simulink model "control_system"  (R2019b)
settings: Solver=FixedStepAuto  StartTime=0.0  StopTime=10.0  RelTol=1e-3
undefined symbols (not defined in the file): thrust_lower_limit, thrust_upper_limit
settings Model: Creator=logan  LastModifiedBy=loganfillo
settings OptimizationCC: DefaultParameterBehavior=Inlined  UseDivisionForNetSlopeComputation=on  GainParamInheritBuiltInType=on  UseFloatMulNetSlope=on  InlineInvariantSignals=on  PassReuseOutputArgsAs=Individual arguments  ZeroExternalMemoryAtStartup=off  ZeroInternalMemoryAtStartup=off  NoFixptDivByZeroProtection=on  EfficientFloat2IntCast=on  LifeSpan=1  OptimizeBlockOrder=speed  DifferentSizesBufferReuse=on  EfficientTunableParamExpr=on
settings DebuggingCC: ParameterTunabilityLossMsg=error
settings HardwareCC: ProdLongLongMode=on
settings SFSimCC: MATLABDynamicMemAlloc=off
settings RTWCC: SystemTargetFile=ert.tlc  PackageGeneratedCodeAndArtifacts=on  TemplateMakefile=ert_default_tmf  GenerateReport=on  IncludeHyperlinkInReport=on  LaunchReport=on  TargetLang=C++  GenerateTraceInfo=on  GenerateTraceReport=on  GenerateTraceReportSl=on  GenerateTraceReportSf=on  GenerateTraceReportEml=on
settings CodeAppCC: ForceParamTrailComments=on  IgnoreCustomStorageClasses=off  OperatorAnnotations=on  SimulinkDataObjDesc=on  SFDataObjDesc=on  InsertBlockDesc=on
settings ERTTargetCC: TargetLangStandard=C++03 (ISO)  GenerateSampleERTMain=on  IncludeMdlTerminateFcn=off  CombineSignalStateStructs=on  MultiInstanceERTCode=on  CodeInterfacePackaging=C++ class  SupportComplex=off  SupportContinuousTime=on  InlinedParameterPlacement=NonHierarchical  RootIOFormat=Structure reference  ERTCustomFileTemplate=example_file_process.tlc  ERTFilePackagingFormat=CompactWithDataFile

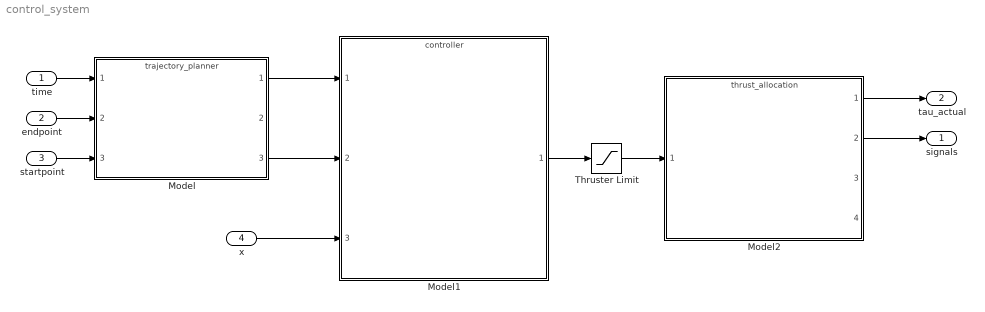
== system control_system ==
  "time " : Inport
  "endpoint " : Inport  Port=2  PortDimensions=6
  startpoint : Inport  Port=3  PortDimensions=6
  x : Inport  Port=4
  Model : ModelReference  ModelNameDialog=trajectory_planner.slx  SimulationMode=Normal  ModelReferenceVersion=1.30
  Model1 : ModelReference  ModelNameDialog=controller.slx  SimulationMode=Normal  ModelReferenceVersion=1.73
  Model2 : ModelReference  ModelNameDialog=thrust_allocation.slx  SimulationMode=Normal  ModelReferenceVersion=1.76
  Thruster Limit : Saturate  UpperLimit=thrust_upper_limit  LowerLimit=thrust_lower_limit
  signals : Outport  VectorParamsAs1DForOutWhenUnconnected=off
  tau_actual : Outport  Port=2
  wires:
  "time "/1 -> Model/1
  "endpoint "/1 -> Model/2
  Model/1 -> Model1/1
  Model1/1 -> Thruster Limit/1
  x/1 -> Model1/3
  Model2/2 -> signals/1
  Thruster Limit/1 -> Model2/1
  Model2/1 -> tau_actual/1
  Model/3 -> Model1/2
  startpoint/1 -> Model/3
